simulink model "rectifiers01"  (R2020b)
settings: Solver=VariableStepAuto  StartTime=0.0  StopTime=2/60  RelTol=1e-3
InitFcn:
  | R = 1;
libraries: fl_lib x61, ee_lib x29, nesl_utility x28, powerlib x1
settings Model: Creator=gdudgeon  LastModifiedBy=gdudgeon
settings DataIOCC: SaveOutput=off  DSMLogging=off  InspectSignalLogs=on  SaveTime=off  ReturnWorkspaceOutputs=off

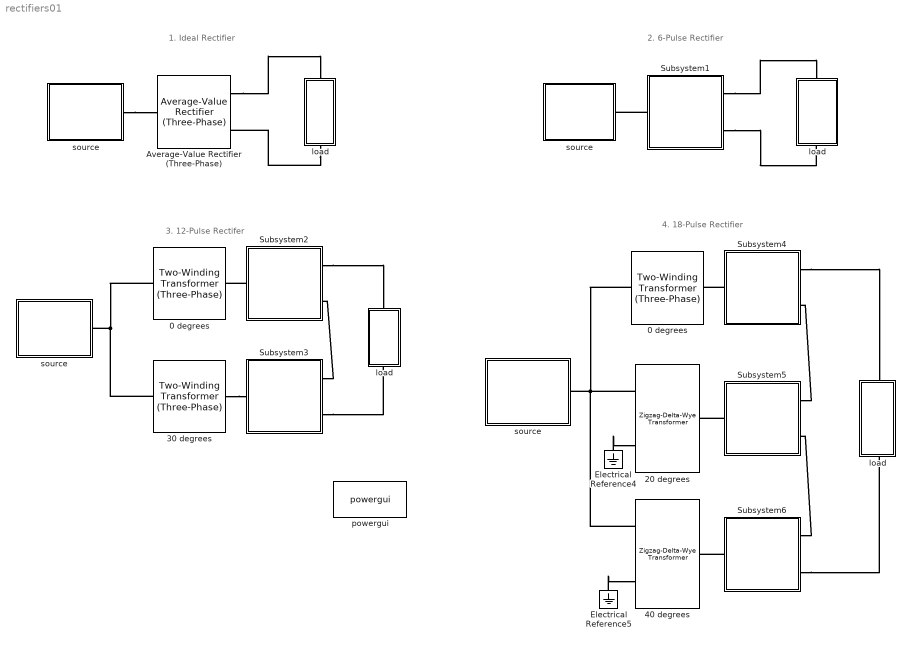
== system rectifiers01 ==
  note: 4. 18-Pulse Rectifier
  note: 3. 12-Pulse Rectifer
  note: 2. 6-Pulse Rectifier
  note: 1. Ideal Rectifier
  " load" : Subsystem
      settings: PortSchema="{\"entries\":[{\"content\":{\"sides\":[{\"content\":{\"connectorIds\":[]},\"type\":\"ConnectorPlacement.EquallySpacedRectSide\",\"uuid\":\"d22d21fe-0203-4dc0-90b3-23bdd03d5351\"},{\"content\":{\"connectorIds\":[],\"side\":\"RIGHT\"},\"type\":\"ConnectorPlacement.EquallySpacedRectSide\",\"uuid\":\"b0134291-2b85-4d9d-ab7a-f2a22f0cc825\"},{\"content\":{\"connectorIds\":[\"LConn1\"],\"side\":\"TOP\"},\"type\":\"ConnectorPlacement.EquallySpacedRectSide\",\"uuid\":\"0f25709f-cbaa-4d6a-91aa-03a240b6065b\"},{\"content\":{\"connectorIds\":[\"RConn1\"],\"side\":\"BOTTOM\"},\"type\":\"ConnectorPlacement.EquallySpacedRectSide\",\"uuid\":\"1cb50f91-b6f6-42a0-b153-9b586f859798\"},{\"content\":{\"connectorIds\":[],\"side\":\"HIDDEN\"},\"type\":\"ConnectorPlacement.EquallySpacedRectSide\",\"uuid\":\"613bd7c7-2abb-4a7f-9569-314c864fd2f9\"}]},\"type\":\"ConnectorPlacement.EquallySpacedConnector\",\"uuid\":\"0347b9d2-0f82-406a-989b-2d0201140953\"}],\"packageUris\":[\"http://schema.mathworks.com/mf0/Connector/R2020b\"],\"version\":\"1.0\"}"
  " source" : Subsystem
  0 degrees : ee_lib/Passive/Transformers/Two-Winding Transformer (Three-Phase)  SRated=100e3 V*A  FRated=60 Hz  Winding1Connection=ee.enum.windingconnection.Y  VRated1=sqrt(3) * 100 / sqrt(2) V  Winding2Connection=ee.enum.windingconnection.Y  VRated2=sqrt(3) * 50 / sqrt(2) V  CoreType=ee.enum.coretype.threelimb  pu_Rw1=0.01e-3  pu_Xl1=0.001e-3  pu_Rw2=0.01e-3  pu_Xl2=0.001e-3  pu_Rm=50000  saturation_option=ee.enum.transformer_saturation.exclude  pu_Xm=50000  current_data=[0, .002, 1, 2]  magnetic_flux_data=[0, 1.2, 1.5, 1.51]  pu_X0=0.5  i1_specify=off  i1_priority=None  i1=[ 0 0 0 ] A  i1_nominal_specify=off  i1_nominal_unit=A  i1_nominal_value=1  i2_specify=off  i2_priority=None  i2=[ 0 0 0 ] A  i2_nominal_specify=off  i2_nominal_unit=A  i2_nominal_value=1  phi_specify=off  phi_priority=None  phi=[ 0 0 0 ]  phi_nominal_specify=off  phi_nominal_unit=1  phi_nominal_value=1  power_dissipated_specify=off  power_dissipated_priority=None  power_dissipated=0 W  power_dissipated_nominal_specify=off  power_dissipated_nominal_unit=W  power_dissipated_nominal_value=1
      settings: SourceProductBaseCode=PS  InternalSimscapePortConfiguration="{\"Bottom\":[],\"Left\":[{\"id\":\"N1\",\"label\":\"~1\",\"type\":\"foundation.electrical.three_phase\"}],\"Right\":[{\"id\":\"N2\",\"label\":\"~2\",\"type\":\"foundation.electrical.three_phase\"}],\"Top\":[]}"
  "0 degrees " : ee_lib/Passive/Transformers/Two-Winding Transformer (Three-Phase)  SRated=100e3 V*A  FRated=60 Hz  Winding1Connection=ee.enum.windingconnection.Y  VRated1=sqrt(3) * 100 / sqrt(2) V  Winding2Connection=ee.enum.windingconnection.Y  VRated2=sqrt(3) * 33.3 / sqrt(2) V  CoreType=ee.enum.coretype.threelimb  pu_Rw1=0.01e-3  pu_Xl1=0.001e-3  pu_Rw2=0.01e-3  pu_Xl2=0.001e-3  pu_Rm=50000  saturation_option=ee.enum.transformer_saturation.exclude  pu_Xm=50000  current_data=[0, .002, 1, 2]  magnetic_flux_data=[0, 1.2, 1.5, 1.51]  pu_X0=0.5  i1_specify=off  i1_priority=None  i1=[ 0 0 0 ] A  i1_nominal_specify=off  i1_nominal_unit=A  i1_nominal_value=1  i2_specify=off  i2_priority=None  i2=[ 0 0 0 ] A  i2_nominal_specify=off  i2_nominal_unit=A  i2_nominal_value=1  phi_specify=off  phi_priority=None  phi=[ 0 0 0 ]  phi_nominal_specify=off  phi_nominal_unit=1  phi_nominal_value=1  power_dissipated_specify=off  power_dissipated_priority=None  power_dissipated=0 W  power_dissipated_nominal_specify=off  power_dissipated_nominal_unit=W  power_dissipated_nominal_value=1
      settings: SourceProductBaseCode=PS  InternalSimscapePortConfiguration="{\"Bottom\":[],\"Left\":[{\"id\":\"N1\",\"label\":\"~1\",\"type\":\"foundation.electrical.three_phase\"}],\"Right\":[{\"id\":\"N2\",\"label\":\"~2\",\"type\":\"foundation.electrical.three_phase\"}],\"Top\":[]}"
  20 degrees : ee_lib/Passive/Transformers/Zigzag-Delta-Wye Transformer  SRated=100e3 V*A  FRated=60 Hz  VRated1=sqrt(3) * 33.3 / sqrt(2) V  interconnection_option=ee.enum.zigzaginterconnection.floatingNeutral  configuration_option=ee.enum.zigzagconfiguration.Wye  pu_Rw1=0.01e-3  pu_Xl1=0.001e-3  pu_Rm=50000  saturation_option=ee.enum.transformer_saturation.exclude  deltaconnection_option=ee.enum.deltaconnection.delta1  VRated2=sqrt(3) * 50 / sqrt(2) V  magnetic_flux_data=[0, 1.2, 1.5, 1.51]  pu_Rw2=0.01  pu_Xl2=0.001  VRated3=sqrt(3) * 100 / sqrt(2) V  pu_Rw3=0.01e-3  pu_Xl3=0.001e-3  pu_Xm=50000  current_data=[0, .002, 1, 2]  phaseShift=20 deg  i1_specify=off  i1_priority=None  i1=[ 0 0 0 ] A  i1_nominal_specify=off  i1_nominal_unit=A  i1_nominal_value=1  i2_specify=off  i2_priority=None  i2=[ 0 0 0 ] A  i2_nominal_specify=off  i2_nominal_unit=A  i2_nominal_value=1  i3_specify=off  i3_priority=None  i3=[ 0 0 0 ] A  i3_nominal_specify=off  i3_nominal_unit=A  i3_nominal_value=1  phi_specify=off  phi_priority=None  phi=[ 0 0 0 ]  phi_nominal_specify=off  phi_nominal_unit=1  phi_nominal_value=1  phaseShift_increment=0.1 deg
      settings: SourceProductBaseCode=PS  InternalSimscapePortConfiguration="{\"Bottom\":[],\"Left\":[{\"id\":\"N1\",\"label\":\"~1\",\"type\":\"foundation.electrical.three_phase\"}],\"Right\":[{\"id\":\"N3\",\"label\":\"~3\",\"type\":\"foundation.electrical.three_phase\"},{\"id\":\"n3\",\"label\":\"n3\",\"type\":\"foundation.electrical.electrical\"}],\"Top\":[]}"
  30 degrees : ee_lib/Passive/Transformers/Two-Winding Transformer (Three-Phase)  SRated=100e3 V*A  FRated=60 Hz  Winding1Connection=ee.enum.windingconnection.delta1  VRated1=sqrt(3) * 100 / sqrt(2) V  Winding2Connection=ee.enum.windingconnection.Y  VRated2=sqrt(3) * 50 / sqrt(2) V  CoreType=ee.enum.coretype.threelimb  pu_Rw1=0.01e-3  pu_Xl1=0.001e-3  pu_Rw2=0.01e-3  pu_Xl2=0.001e-3  pu_Rm=50000  saturation_option=ee.enum.transformer_saturation.exclude  pu_Xm=50000  current_data=[0, .002, 1, 2]  magnetic_flux_data=[0, 1.2, 1.5, 1.51]  pu_X0=0.5  i1_specify=off  i1_priority=None  i1=[ 0 0 0 ] A  i1_nominal_specify=off  i1_nominal_unit=A  i1_nominal_value=1  i2_specify=off  i2_priority=None  i2=[ 0 0 0 ] A  i2_nominal_specify=off  i2_nominal_unit=A  i2_nominal_value=1  phi_specify=off  phi_priority=None  phi=[ 0 0 0 ]  phi_nominal_specify=off  phi_nominal_unit=1  phi_nominal_value=1  power_dissipated_specify=off  power_dissipated_priority=None  power_dissipated=0 W  power_dissipated_nominal_specify=off  power_dissipated_nominal_unit=W  power_dissipated_nominal_value=1
      settings: SourceProductBaseCode=PS  InternalSimscapePortConfiguration="{\"Bottom\":[],\"Left\":[{\"id\":\"N1\",\"label\":\"~1\",\"type\":\"foundation.electrical.three_phase\"}],\"Right\":[{\"id\":\"N2\",\"label\":\"~2\",\"type\":\"foundation.electrical.three_phase\"}],\"Top\":[]}"
  40 degrees : ee_lib/Passive/Transformers/Zigzag-Delta-Wye Transformer  SRated=100e3 V*A  FRated=60 Hz  VRated1=sqrt(3) * 33.3 / sqrt(2) V  interconnection_option=ee.enum.zigzaginterconnection.floatingNeutral  configuration_option=ee.enum.zigzagconfiguration.Wye  pu_Rw1=0.01e-3  pu_Xl1=0.001e-3  pu_Rm=50000  saturation_option=ee.enum.transformer_saturation.exclude  deltaconnection_option=ee.enum.deltaconnection.delta1  VRated2=sqrt(3) * 50 / sqrt(2) V  magnetic_flux_data=[0, 1.2, 1.5, 1.51]  pu_Rw2=0.01  pu_Xl2=0.001  VRated3=sqrt(3) * 100 / sqrt(2) V  pu_Rw3=0.01e-3  pu_Xl3=0.001e-3  pu_Xm=50000  current_data=[0, .002, 1, 2]  phaseShift=40 deg  i1_specify=off  i1_priority=None  i1=[ 0 0 0 ] A  i1_nominal_specify=off  i1_nominal_unit=A  i1_nominal_value=1  i2_specify=off  i2_priority=None  i2=[ 0 0 0 ] A  i2_nominal_specify=off  i2_nominal_unit=A  i2_nominal_value=1  i3_specify=off  i3_priority=None  i3=[ 0 0 0 ] A  i3_nominal_specify=off  i3_nominal_unit=A  i3_nominal_value=1  phi_specify=off  phi_priority=None  phi=[ 0 0 0 ]  phi_nominal_specify=off  phi_nominal_unit=1  phi_nominal_value=1  phaseShift_increment=0.1 deg
      settings: SourceProductBaseCode=PS  InternalSimscapePortConfiguration="{\"Bottom\":[],\"Left\":[{\"id\":\"N1\",\"label\":\"~1\",\"type\":\"foundation.electrical.three_phase\"}],\"Right\":[{\"id\":\"N3\",\"label\":\"~3\",\"type\":\"foundation.electrical.three_phase\"},{\"id\":\"n3\",\"label\":\"n3\",\"type\":\"foundation.electrical.electrical\"}],\"Top\":[]}"
  Average-Value Rectifier (Three-Phase) : ee_lib/Semiconductors & Converters/Converters/Average-Value Rectifier (Three-Phase)  VRated=4160 V  Pfixed=1e3 W
      settings: SourceProductBaseCode=PS  InternalSimscapePortConfiguration="{\"Bottom\":[],\"Left\":[{\"id\":\"N\",\"label\":\"~\",\"type\":\"foundation.electrical.three_phase\"}],\"Right\":[{\"id\":\"p\",\"label\":\"+\",\"type\":\"foundation.electrical.electrical\"},{\"id\":\"n\",\"label\":\"-\",\"type\":\"foundation.electrical.electrical\"}],\"Top\":[]}"
  Electrical Reference4 : fl_lib/Electrical/Electrical Elements/Electrical Reference
  Electrical Reference5 : fl_lib/Electrical/Electrical Elements/Electrical Reference
  Subsystem1 : Subsystem
      mask Display: image('diode.jpg')
  Subsystem2 : Subsystem
      mask Display: image('diode.jpg')
  Subsystem3 : Subsystem
      mask Display: image('diode.jpg')
  Subsystem4 : Subsystem
      mask Display: image('diode.jpg')
  Subsystem5 : Subsystem
      mask Display: image('diode.jpg')
  Subsystem6 : Subsystem
      mask Display: image('diode.jpg')
  load : Subsystem
      settings: PortSchema="{\"entries\":[{\"content\":{\"sides\":[{\"content\":{\"connectorIds\":[]},\"type\":\"ConnectorPlacement.EquallySpacedRectSide\",\"uuid\":\"d22d21fe-0203-4dc0-90b3-23bdd03d5351\"},{\"content\":{\"connectorIds\":[],\"side\":\"RIGHT\"},\"type\":\"ConnectorPlacement.EquallySpacedRectSide\",\"uuid\":\"b0134291-2b85-4d9d-ab7a-f2a22f0cc825\"},{\"content\":{\"connectorIds\":[\"LConn1\"],\"side\":\"TOP\"},\"type\":\"ConnectorPlacement.EquallySpacedRectSide\",\"uuid\":\"0f25709f-cbaa-4d6a-91aa-03a240b6065b\"},{\"content\":{\"connectorIds\":[\"RConn1\"],\"side\":\"BOTTOM\"},\"type\":\"ConnectorPlacement.EquallySpacedRectSide\",\"uuid\":\"adaf0646-c50e-4c15-9e13-216df2ff67a6\"},{\"content\":{\"connectorIds\":[],\"side\":\"HIDDEN\"},\"type\":\"ConnectorPlacement.EquallySpacedRectSide\",\"uuid\":\"613bd7c7-2abb-4a7f-9569-314c864fd2f9\"}]},\"type\":\"ConnectorPlacement.EquallySpacedConnector\",\"uuid\":\"0347b9d2-0f82-406a-989b-2d0201140953\"}],\"packageUris\":[\"http://schema.mathworks.com/mf0/Connector/R2020b\"],\"version\":\"1.0\"}"
  "load " : Subsystem
      settings: PortSchema="{\"entries\":[{\"content\":{\"sides\":[{\"content\":{\"connectorIds\":[]},\"type\":\"ConnectorPlacement.EquallySpacedRectSide\",\"uuid\":\"d22d21fe-0203-4dc0-90b3-23bdd03d5351\"},{\"content\":{\"connectorIds\":[],\"side\":\"RIGHT\"},\"type\":\"ConnectorPlacement.EquallySpacedRectSide\",\"uuid\":\"b0134291-2b85-4d9d-ab7a-f2a22f0cc825\"},{\"content\":{\"connectorIds\":[\"LConn1\"],\"side\":\"TOP\"},\"type\":\"ConnectorPlacement.EquallySpacedRectSide\",\"uuid\":\"0f25709f-cbaa-4d6a-91aa-03a240b6065b\"},{\"content\":{\"connectorIds\":[\"RConn1\"],\"side\":\"BOTTOM\"},\"type\":\"ConnectorPlacement.EquallySpacedRectSide\",\"uuid\":\"28ce9175-6449-4b65-9253-b55dcacbce87\"},{\"content\":{\"connectorIds\":[],\"side\":\"HIDDEN\"},\"type\":\"ConnectorPlacement.EquallySpacedRectSide\",\"uuid\":\"613bd7c7-2abb-4a7f-9569-314c864fd2f9\"}]},\"type\":\"ConnectorPlacement.EquallySpacedConnector\",\"uuid\":\"0347b9d2-0f82-406a-989b-2d0201140953\"}],\"packageUris\":[\"http://schema.mathworks.com/mf0/Connector/R2020b\"],\"version\":\"1.0\"}"
  "load  " : Subsystem
      settings: PortSchema="{\"entries\":[{\"content\":{\"sides\":[{\"content\":{\"connectorIds\":[]},\"type\":\"ConnectorPlacement.EquallySpacedRectSide\",\"uuid\":\"d22d21fe-0203-4dc0-90b3-23bdd03d5351\"},{\"content\":{\"connectorIds\":[],\"side\":\"RIGHT\"},\"type\":\"ConnectorPlacement.EquallySpacedRectSide\",\"uuid\":\"b0134291-2b85-4d9d-ab7a-f2a22f0cc825\"},{\"content\":{\"connectorIds\":[\"LConn1\"],\"side\":\"TOP\"},\"type\":\"ConnectorPlacement.EquallySpacedRectSide\",\"uuid\":\"0f25709f-cbaa-4d6a-91aa-03a240b6065b\"},{\"content\":{\"connectorIds\":[\"RConn1\"],\"side\":\"BOTTOM\"},\"type\":\"ConnectorPlacement.EquallySpacedRectSide\",\"uuid\":\"e9fa62c1-7df6-4db7-8279-90334c7dd692\"},{\"content\":{\"connectorIds\":[],\"side\":\"HIDDEN\"},\"type\":\"ConnectorPlacement.EquallySpacedRectSide\",\"uuid\":\"613bd7c7-2abb-4a7f-9569-314c864fd2f9\"}]},\"type\":\"ConnectorPlacement.EquallySpacedConnector\",\"uuid\":\"0347b9d2-0f82-406a-989b-2d0201140953\"}],\"packageUris\":[\"http://schema.mathworks.com/mf0/Connector/R2020b\"],\"version\":\"1.0\"}"
  powergui : powerlib/powergui  Priority=1  SimulationMode=Continuous  SampleTime=50e-6  frequency=60  Iterations=50  frequencyindice=60  Pbase=100e6  ErrMax=1e-4  UnitsV=kV  UnitsW=MW  buscounter=0  FunctionMessages=off  echomessages=off  EnableUseOfTLC=off  CurrentSourceSwitches=off  DisableSnubberDevices=off  DisableRonSwitches=off  DisableVfSwitches=off  DisplayEquations=off  AutomaticDiscreteSolvers=off  SolverType=Tustin/Backward Euler (TBE)  Interpol=off  ExternalGateDelay=off  methode=off  Ts=100  x0status=blocks  SPID=on  SwTol=0  HookPort=off  NonlinearTolerance=1e-4  nMaxIteration=100  ContinueOnMaxIteration=off  RestoreLinks=warning  ResistiveCurrentMeasurement=off  Frange=[0:2:500]  Ylog=off  Xlog=on  ShowGrid=off  save=off  variable=ZData  structure=logsout  ZoomFFT=off  StartTime=0.01  cycles=1  DisplayStyle=1  fundamental=60  FreqAxis=on  MaxFrequency=2000  frequencyindicesteady=1  RmsSteady=1  display=off
  source : Subsystem
  "source " : Subsystem
  "source  " : Subsystem
  connections:
  Subsystem3/LConn1 -- Subsystem2/LConn2
  30 degrees/RConn1 -- Subsystem3/RConn1
  Subsystem2/RConn1 -- 0 degrees/RConn1
  Subsystem4/RConn1 -- "0 degrees "/RConn1
  Subsystem5/LConn1 -- Subsystem4/LConn2
  Subsystem5/RConn1 -- 20 degrees/LConn1
  Electrical Reference4/LConn1 -- 20 degrees/RConn2
  Subsystem6/RConn1 -- 40 degrees/LConn1
  Electrical Reference5/LConn1 -- 40 degrees/RConn2
  Subsystem6/LConn1 -- Subsystem5/LConn2
  source/RConn1 -- Average-Value Rectifier (Three-Phase)/LConn1
  Average-Value Rectifier (Three-Phase)/RConn1 -- load/LConn1
  load/RConn1 -- Average-Value Rectifier (Three-Phase)/RConn2
  Subsystem2/LConn1 -- "load "/LConn1
  Subsystem3/LConn2 -- "load "/RConn1
  0 degrees/LConn1 -- 30 degrees/LConn1 -- "source "/RConn1
  Subsystem1/RConn1 -- "source  "/RConn1
  Subsystem1/LConn1 -- "load  "/LConn1
  Subsystem1/LConn2 -- "load  "/RConn1
  20 degrees/RConn1 -- "0 degrees "/LConn1 -- 40 degrees/RConn1 -- " source"/RConn1
  Subsystem4/LConn1 -- " load"/LConn1
  Subsystem6/LConn2 -- " load"/RConn1

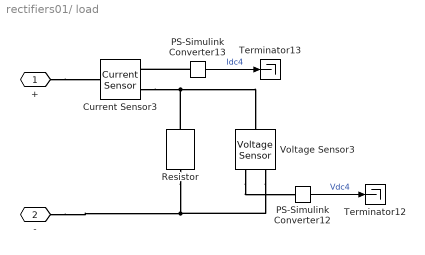
== system rectifiers01/ load ==
  Current Sensor3 : fl_lib/Electrical/Electrical Sensors/Current Sensor
  PS-Simulink Converter12 : nesl_utility/PS-Simulink Converter  PhysicalDomain=network_engine_domain  SubClassName=ps_output  LeftPortType=input  RightPortType=output  PseudoPeriodic=off  Frequencies=[]  Unit=inherit  AffineConversion=off
  PS-Simulink Converter13 : nesl_utility/PS-Simulink Converter  PhysicalDomain=network_engine_domain  SubClassName=ps_output  LeftPortType=input  RightPortType=output  PseudoPeriodic=off  Frequencies=[]  Unit=inherit  AffineConversion=off
  Resistor : fl_lib/Electrical/Electrical Elements/Resistor  R=R Ohm  i_specify=off  i_priority=None  i=0 A  i_nominal_specify=off  i_nominal_unit=A  i_nominal_value=1  v_specify=off  v_priority=None  v=0 V  v_nominal_specify=off  v_nominal_unit=V  v_nominal_value=1
  Terminator12 : Terminator
  Terminator13 : Terminator
  Voltage Sensor3 : fl_lib/Electrical/Electrical Sensors/Voltage Sensor
  + : PMIOPort  Side=Left
  - : PMIOPort  Port=2  Side=Right
  wires:
  PS-Simulink Converter13/1 -> Terminator13/1  "Idc4"
  PS-Simulink Converter12/1 -> Terminator12/1  "Vdc4"
  connections:
  +/RConn1 -- Current Sensor3/LConn1
  Voltage Sensor3/RConn1 -- PS-Simulink Converter12/LConn1
  Current Sensor3/RConn2 -- Resistor/LConn1 -- Voltage Sensor3/LConn1
  PS-Simulink Converter13/LConn1 -- Current Sensor3/RConn1
  Voltage Sensor3/RConn2 -- Resistor/RConn1 -- -/RConn1

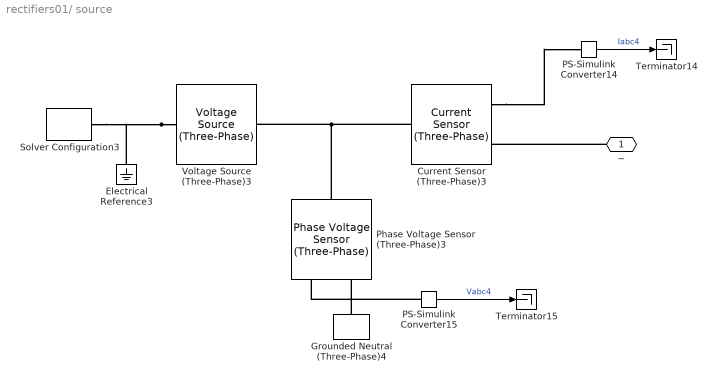
== system rectifiers01/ source ==
  Current Sensor (Three-Phase)3 : ee_lib/Sensors & Transducers/Current Sensor (Three-Phase)
  Electrical Reference3 : fl_lib/Electrical/Electrical Elements/Electrical Reference
  Grounded Neutral (Three-Phase)4 : ee_lib/Connectors & References/Grounded Neutral (Three-Phase)
      settings: SourceProductBaseCode=PS
  PS-Simulink Converter14 : nesl_utility/PS-Simulink Converter  PhysicalDomain=network_engine_domain  SubClassName=ps_output  LeftPortType=input  RightPortType=output  PseudoPeriodic=off  Frequencies=[]  Unit=inherit  AffineConversion=off
  PS-Simulink Converter15 : nesl_utility/PS-Simulink Converter  PhysicalDomain=network_engine_domain  SubClassName=ps_output  LeftPortType=input  RightPortType=output  PseudoPeriodic=off  Frequencies=[]  Unit=inherit  AffineConversion=off
  Phase Voltage Sensor (Three-Phase)3 : ee_lib/Sensors & Transducers/Phase Voltage Sensor (Three-Phase)
      settings: SourceProductBaseCode=PS
  Solver Configuration3 : nesl_utility/Solver Configuration  PhysicalDomain=network_engine_domain  SubClassName=solver  LeftPortType=input  RightPortType=generic  Tones=[]  Harmonics=[]  SimulateNoise=off  Profile=off  UseLocalSampling=off  EnableSwitchedLinearOptims=on  FrequencyDomain=off  UseCCode=off  RelTol=0.001  AbsTol=1e-06  MinStep=1e-09  ToWorkspace=off  RevertToSquareIcSolve=off  NumHomotopyIterations=100  PhasorMode=off  PhasorModeNumHarmonics=1  DoDC=off  ResidualTolerance=1e-09  UseLocalSolver=on  LocalSolverChoice=NE_BACKWARD_EULER_ADVANCER  LocalSolverSampleTime=50e-6  DoFixedCost=on  MaxNonlinIter=3  MaxModeIter=2  ComputeImpulses=off  ImpulseIterations=2  LinearAlgebra=auto  EquationFormulation=NE_TIME_EF  DelaysMemoryBudget=1024  AutomaticFiltering=on  FilteringTimeConstant=0.001  PartitionStorageMethod=AS_NEEDED  PartitionMemoryBudget=1024  PartitionMethod=ROBUST
  Terminator14 : Terminator
  Terminator15 : Terminator
  Voltage Source (Three-Phase)3 : ee_lib/Sources/Voltage Source (Three-Phase)  vline_rms=sqrt(3) * 100 / sqrt(2) V  shift=0 deg  freq=60 Hz  impedance_option=0  SShortCircuit=1e6 V*A  XR=15  R=0.01 Ohm  L=3.97e-4 H  G_parasitic=0 1/Ohm  harmonic_option=0  harmonic_orders=[5, 7, 11, 13]  harmonic_ratios=[.1, .1, .1, .1]  I_specify=off  I_priority=None  I=[ 0 0 0 ] A  I_nominal_specify=off  I_nominal_unit=A  I_nominal_value=1
      settings: SourceProductBaseCode=PS
  ~ : PMIOPort  Side=Right
  wires:
  PS-Simulink Converter15/1 -> Terminator15/1  "Vabc4"
  PS-Simulink Converter14/1 -> Terminator14/1  "Iabc4"
  connections:
  Grounded Neutral (Three-Phase)4/LConn1 -- Phase Voltage Sensor (Three-Phase)3/RConn2
  Current Sensor (Three-Phase)3/RConn1 -- PS-Simulink Converter14/LConn1
  Phase Voltage Sensor (Three-Phase)3/LConn1 -- Current Sensor (Three-Phase)3/LConn1 -- Voltage Source (Three-Phase)3/RConn1
  PS-Simulink Converter15/LConn1 -- Phase Voltage Sensor (Three-Phase)3/RConn1
  Voltage Source (Three-Phase)3/LConn1 -- Electrical Reference3/LConn1 -- Solver Configuration3/RConn1
  ~/RConn1 -- Current Sensor (Three-Phase)3/RConn2

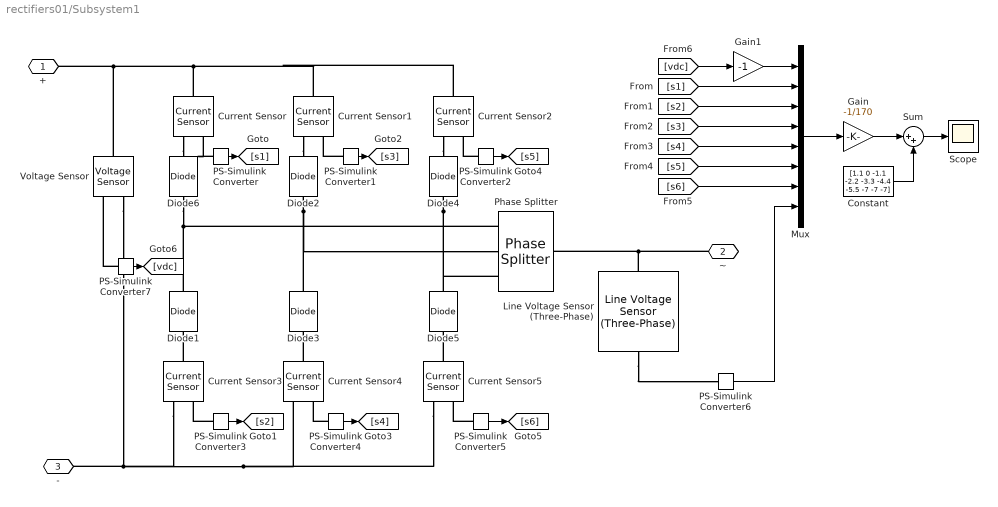
== system rectifiers01/Subsystem1 ==
  Constant : Constant  Value=[1.1 0 -1.1 -2.2 -3.3 -4.4 -5.5 -7 -7 -7]
  Current Sensor{,1..5} (6 alike) : fl_lib/Electrical/Electrical Sensors/Current Sensor
  Diode{1..6} (6 alike) : fl_lib/Electrical/Electrical Elements/Diode  Vf=0.6 V  Ron=1e-5 Ohm  Goff=1e-8 1/Ohm  i_specify=off  i_priority=None  i=0 A  i_nominal_specify=off  i_nominal_unit=A  i_nominal_value=1  v_specify=off  v_priority=None  v=0 V  v_nominal_specify=off  v_nominal_unit=V  v_nominal_value=1
  Gain : Gain  Gain=-1/170
  Gain1 : Gain  Gain=-1
  Line Voltage Sensor (Three-Phase) : ee_lib/Sensors & Transducers/Line Voltage Sensor (Three-Phase)
      settings: SourceProductBaseCode=PS
  Mux : Mux  Inputs=8
  PS-Simulink Converter{,1..7} (8 alike) : nesl_utility/PS-Simulink Converter  PhysicalDomain=network_engine_domain  SubClassName=ps_output  LeftPortType=input  RightPortType=output  PseudoPeriodic=off  Frequencies=[]  Unit=inherit  AffineConversion=off
  Phase Splitter : ee_lib/Connectors & References/Phase Splitter
      settings: SourceProductBaseCode=PS
  Scope : Scope
  Sum : Sum  Inputs=|++
  Voltage Sensor : fl_lib/Electrical/Electrical Sensors/Voltage Sensor
  + : PMIOPort  Side=Left
  ~ : PMIOPort  Port=2  Side=Right
  - : PMIOPort  Port=3  Side=Left
  wires:
  PS-Simulink Converter/1 -> [s1]
  PS-Simulink Converter3/1 -> [s2]
  PS-Simulink Converter1/1 -> [s3]
  PS-Simulink Converter4/1 -> [s4]
  PS-Simulink Converter2/1 -> [s5]
  PS-Simulink Converter5/1 -> [s6]
  Mux/1 -> Gain/1
  Gain/1 -> Sum/1
  Sum/1 -> Scope/1
  Constant/1 -> Sum/2
  PS-Simulink Converter6/1 -> Mux/8
  PS-Simulink Converter7/1 -> [vdc]
  [vdc] -> Gain1/1
  [s1] -> Mux/2
  [s2] -> Mux/3
  [s3] -> Mux/4
  [s4] -> Mux/5
  [s5] -> Mux/6
  [s6] -> Mux/7
  Gain1/1 -> Mux/1
  connections:
  Diode4/LConn1 -- Phase Splitter/RConn3 -- Diode5/RConn1
  Current Sensor5/RConn2 -- Current Sensor4/RConn2 -- Current Sensor3/RConn2 -- Voltage Sensor/RConn2 -- -/RConn1
  Diode6/LConn1 -- Diode1/RConn1 -- Phase Splitter/RConn1
  Diode2/LConn1 -- Diode3/RConn1 -- Phase Splitter/RConn2
  ~/RConn1 -- Line Voltage Sensor (Three-Phase)/LConn1 -- Phase Splitter/LConn1
  Current Sensor2/LConn1 -- Current Sensor1/LConn1 -- Current Sensor/LConn1 -- Voltage Sensor/LConn1 -- +/RConn1
  Current Sensor/RConn2 -- Diode6/RConn1
  Current Sensor1/RConn2 -- Diode2/RConn1
  Current Sensor2/RConn2 -- Diode4/RConn1
  Current Sensor3/LConn1 -- Diode1/LConn1
  Current Sensor4/LConn1 -- Diode3/LConn1
  Current Sensor5/LConn1 -- Diode5/LConn1
  PS-Simulink Converter/LConn1 -- Current Sensor/RConn1
  PS-Simulink Converter1/LConn1 -- Current Sensor1/RConn1
  PS-Simulink Converter2/LConn1 -- Current Sensor2/RConn1
  PS-Simulink Converter3/LConn1 -- Current Sensor3/RConn1
  PS-Simulink Converter4/LConn1 -- Current Sensor4/RConn1
  PS-Simulink Converter5/LConn1 -- Current Sensor5/RConn1
  Line Voltage Sensor (Three-Phase)/RConn1 -- PS-Simulink Converter6/LConn1
  PS-Simulink Converter7/LConn1 -- Voltage Sensor/RConn1

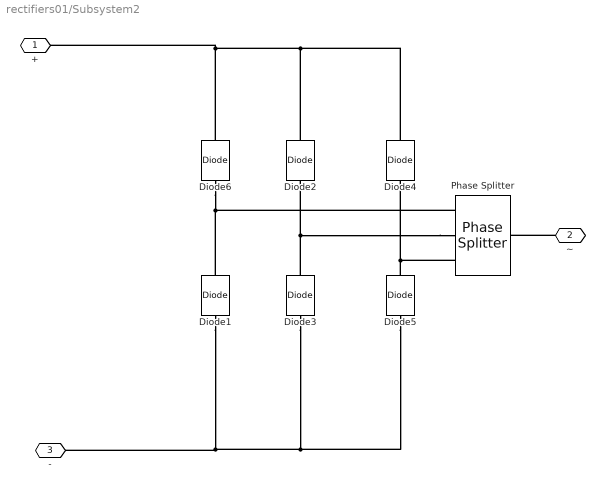
== system rectifiers01/Subsystem2 ==
  Diode{1..6} (6 alike) : fl_lib/Electrical/Electrical Elements/Diode  Vf=0.6 V  Ron=1e-5 Ohm  Goff=1e-8 1/Ohm  i_specify=off  i_priority=None  i=0 A  i_nominal_specify=off  i_nominal_unit=A  i_nominal_value=1  v_specify=off  v_priority=None  v=0 V  v_nominal_specify=off  v_nominal_unit=V  v_nominal_value=1
  Phase Splitter : ee_lib/Connectors & References/Phase Splitter
      settings: SourceProductBaseCode=PS
  + : PMIOPort  Side=Left
  ~ : PMIOPort  Port=2  Side=Right
  - : PMIOPort  Port=3  Side=Left
  connections:
  Diode6/RConn1 -- +/RConn1 -- Diode4/RConn1 -- Diode2/RConn1
  ~/RConn1 -- Phase Splitter/LConn1
  Phase Splitter/RConn2 -- Diode3/RConn1 -- Diode2/LConn1
  Diode1/RConn1 -- Phase Splitter/RConn1 -- Diode6/LConn1
  Diode1/LConn1 -- Diode5/LConn1 -- Diode3/LConn1 -- -/RConn1
  Phase Splitter/RConn3 -- Diode5/RConn1 -- Diode4/LConn1

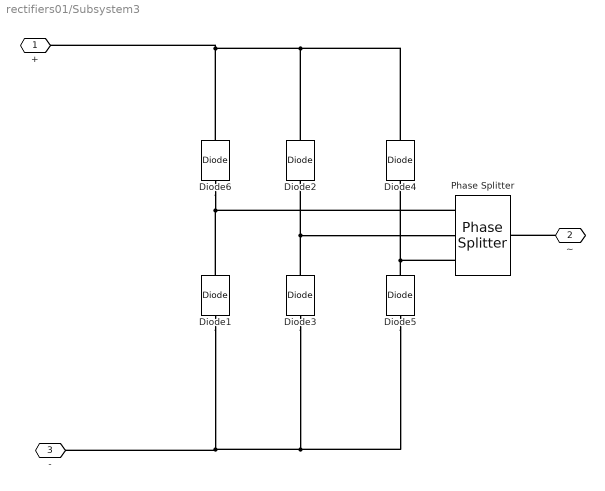
== system rectifiers01/Subsystem3 ==
  Diode{1..6} (6 alike) : fl_lib/Electrical/Electrical Elements/Diode  Vf=0.6 V  Ron=1e-5 Ohm  Goff=1e-8 1/Ohm  i_specify=off  i_priority=None  i=0 A  i_nominal_specify=off  i_nominal_unit=A  i_nominal_value=1  v_specify=off  v_priority=None  v=0 V  v_nominal_specify=off  v_nominal_unit=V  v_nominal_value=1
  Phase Splitter : ee_lib/Connectors & References/Phase Splitter
      settings: SourceProductBaseCode=PS
  + : PMIOPort  Side=Left
  ~ : PMIOPort  Port=2  Side=Right
  - : PMIOPort  Port=3  Side=Left
  connections:
  Diode4/LConn1 -- Diode5/RConn1 -- Phase Splitter/RConn3
  -/RConn1 -- Diode3/LConn1 -- Diode5/LConn1 -- Diode1/LConn1
  Diode6/LConn1 -- Phase Splitter/RConn1 -- Diode1/RConn1
  Diode2/LConn1 -- Diode3/RConn1 -- Phase Splitter/RConn2
  ~/RConn1 -- Phase Splitter/LConn1
  Diode2/RConn1 -- Diode4/RConn1 -- +/RConn1 -- Diode6/RConn1

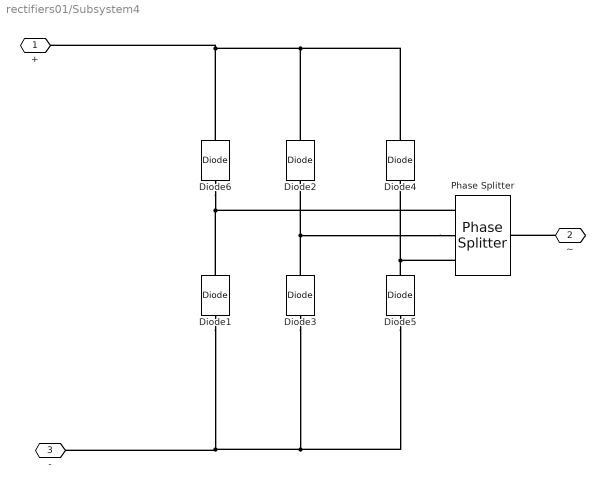
== system rectifiers01/Subsystem4 ==
  Diode{1..6} (6 alike) : fl_lib/Electrical/Electrical Elements/Diode  Vf=0.6 V  Ron=1e-5 Ohm  Goff=1e-8 1/Ohm  i_specify=off  i_priority=None  i=0 A  i_nominal_specify=off  i_nominal_unit=A  i_nominal_value=1  v_specify=off  v_priority=None  v=0 V  v_nominal_specify=off  v_nominal_unit=V  v_nominal_value=1
  Phase Splitter : ee_lib/Connectors & References/Phase Splitter
      settings: SourceProductBaseCode=PS
  + : PMIOPort  Side=Left
  ~ : PMIOPort  Port=2  Side=Right
  - : PMIOPort  Port=3  Side=Left
  connections:
  Diode6/RConn1 -- +/RConn1 -- Diode4/RConn1 -- Diode2/RConn1
  ~/RConn1 -- Phase Splitter/LConn1
  Phase Splitter/RConn2 -- Diode3/RConn1 -- Diode2/LConn1
  Diode1/RConn1 -- Phase Splitter/RConn1 -- Diode6/LConn1
  Diode1/LConn1 -- Diode5/LConn1 -- Diode3/LConn1 -- -/RConn1
  Phase Splitter/RConn3 -- Diode5/RConn1 -- Diode4/LConn1

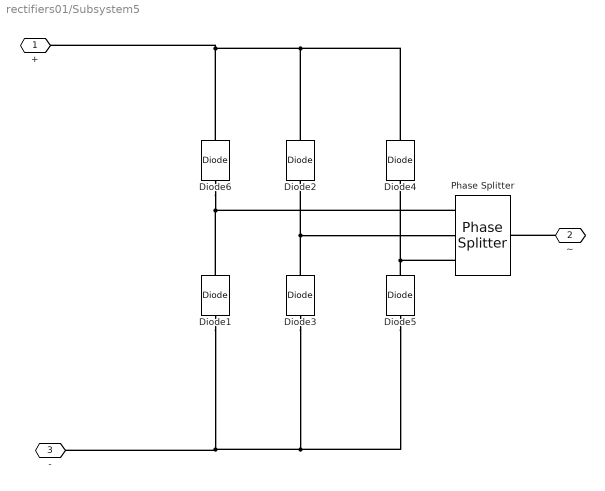
== system rectifiers01/Subsystem5 ==
  Diode{1..6} (6 alike) : fl_lib/Electrical/Electrical Elements/Diode  Vf=0.6 V  Ron=1e-5 Ohm  Goff=1e-8 1/Ohm  i_specify=off  i_priority=None  i=0 A  i_nominal_specify=off  i_nominal_unit=A  i_nominal_value=1  v_specify=off  v_priority=None  v=0 V  v_nominal_specify=off  v_nominal_unit=V  v_nominal_value=1
  Phase Splitter : ee_lib/Connectors & References/Phase Splitter
      settings: SourceProductBaseCode=PS
  + : PMIOPort  Side=Left
  ~ : PMIOPort  Port=2  Side=Right
  - : PMIOPort  Port=3  Side=Left
  connections:
  Diode4/LConn1 -- Diode5/RConn1 -- Phase Splitter/RConn3
  -/RConn1 -- Diode3/LConn1 -- Diode5/LConn1 -- Diode1/LConn1
  Diode6/LConn1 -- Phase Splitter/RConn1 -- Diode1/RConn1
  Diode2/LConn1 -- Diode3/RConn1 -- Phase Splitter/RConn2
  ~/RConn1 -- Phase Splitter/LConn1
  Diode2/RConn1 -- Diode4/RConn1 -- +/RConn1 -- Diode6/RConn1

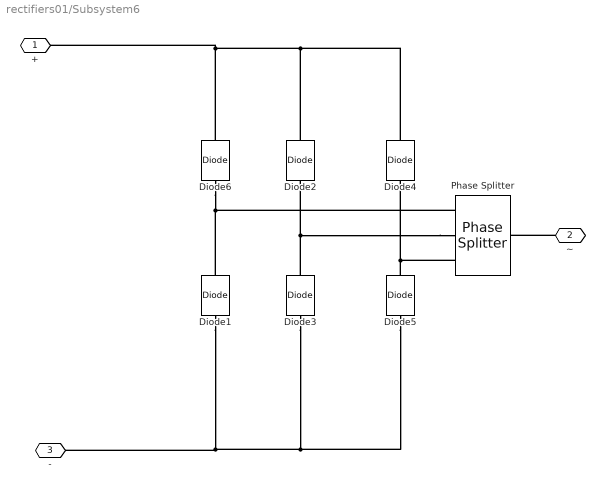
== system rectifiers01/Subsystem6 ==
  Diode{1..6} (6 alike) : fl_lib/Electrical/Electrical Elements/Diode  Vf=0.6 V  Ron=1e-5 Ohm  Goff=1e-8 1/Ohm  i_specify=off  i_priority=None  i=0 A  i_nominal_specify=off  i_nominal_unit=A  i_nominal_value=1  v_specify=off  v_priority=None  v=0 V  v_nominal_specify=off  v_nominal_unit=V  v_nominal_value=1
  Phase Splitter : ee_lib/Connectors & References/Phase Splitter
      settings: SourceProductBaseCode=PS
  + : PMIOPort  Side=Left
  ~ : PMIOPort  Port=2  Side=Right
  - : PMIOPort  Port=3  Side=Left
  connections:
  Diode6/RConn1 -- +/RConn1 -- Diode4/RConn1 -- Diode2/RConn1
  ~/RConn1 -- Phase Splitter/LConn1
  Phase Splitter/RConn2 -- Diode3/RConn1 -- Diode2/LConn1
  Diode1/RConn1 -- Phase Splitter/RConn1 -- Diode6/LConn1
  Diode1/LConn1 -- Diode5/LConn1 -- Diode3/LConn1 -- -/RConn1
  Phase Splitter/RConn3 -- Diode5/RConn1 -- Diode4/LConn1

== system rectifiers01/load ==
  Current Sensor : fl_lib/Electrical/Electrical Sensors/Current Sensor
  PS-Simulink Converter2 : nesl_utility/PS-Simulink Converter  PhysicalDomain=network_engine_domain  SubClassName=ps_output  LeftPortType=input  RightPortType=output  PseudoPeriodic=off  Frequencies=[]  Unit=inherit  AffineConversion=off
  PS-Simulink Converter3 : nesl_utility/PS-Simulink Converter  PhysicalDomain=network_engine_domain  SubClassName=ps_output  LeftPortType=input  RightPortType=output  PseudoPeriodic=off  Frequencies=[]  Unit=inherit  AffineConversion=off
  Resistor : fl_lib/Electrical/Electrical Elements/Resistor  R=R Ohm  i_specify=off  i_priority=None  i=0 A  i_nominal_specify=off  i_nominal_unit=A  i_nominal_value=1  v_specify=off  v_priority=None  v=0 V  v_nominal_specify=off  v_nominal_unit=V  v_nominal_value=1
  Terminator2 : Terminator
  Terminator3 : Terminator
  Voltage Sensor : fl_lib/Electrical/Electrical Sensors/Voltage Sensor
  + : PMIOPort  Side=Left
  - : PMIOPort  Port=2  Side=Right
  wires:
  PS-Simulink Converter3/1 -> Terminator3/1  "Idc1"
  PS-Simulink Converter2/1 -> Terminator2/1  "Vdc1"
  connections:
  +/RConn1 -- Current Sensor/LConn1
  Current Sensor/RConn2 -- Resistor/LConn1 -- Voltage Sensor/LConn1
  Voltage Sensor/RConn1 -- PS-Simulink Converter2/LConn1
  PS-Simulink Converter3/LConn1 -- Current Sensor/RConn1
  Voltage Sensor/RConn2 -- Resistor/RConn1 -- -/RConn1

== system rectifiers01/load  ==
  Current Sensor2 : fl_lib/Electrical/Electrical Sensors/Current Sensor
  PS-Simulink Converter10 : nesl_utility/PS-Simulink Converter  PhysicalDomain=network_engine_domain  SubClassName=ps_output  LeftPortType=input  RightPortType=output  PseudoPeriodic=off  Frequencies=[]  Unit=inherit  AffineConversion=off
  PS-Simulink Converter11 : nesl_utility/PS-Simulink Converter  PhysicalDomain=network_engine_domain  SubClassName=ps_output  LeftPortType=input  RightPortType=output  PseudoPeriodic=off  Frequencies=[]  Unit=inherit  AffineConversion=off
  Resistor : fl_lib/Electrical/Electrical Elements/Resistor  R=R Ohm  i_specify=off  i_priority=None  i=0 A  i_nominal_specify=off  i_nominal_unit=A  i_nominal_value=1  v_specify=off  v_priority=None  v=0 V  v_nominal_specify=off  v_nominal_unit=V  v_nominal_value=1
  Terminator10 : Terminator
  Terminator11 : Terminator
  Voltage Sensor2 : fl_lib/Electrical/Electrical Sensors/Voltage Sensor
  + : PMIOPort  Side=Left
  - : PMIOPort  Port=2  Side=Right
  wires:
  PS-Simulink Converter10/1 -> Terminator10/1  "Vdc3"
  PS-Simulink Converter11/1 -> Terminator11/1  "Idc3"
  connections:
  Current Sensor2/RConn2 -- Resistor/LConn1 -- Voltage Sensor2/LConn1
  PS-Simulink Converter11/LConn1 -- Current Sensor2/RConn1
  Voltage Sensor2/RConn1 -- PS-Simulink Converter10/LConn1
  Voltage Sensor2/RConn2 -- Resistor/RConn1 -- -/RConn1
  +/RConn1 -- Current Sensor2/LConn1

== system rectifiers01/load   ==
  Current Sensor1 : fl_lib/Electrical/Electrical Sensors/Current Sensor
  PS-Simulink Converter6 : nesl_utility/PS-Simulink Converter  PhysicalDomain=network_engine_domain  SubClassName=ps_output  LeftPortType=input  RightPortType=output  PseudoPeriodic=off  Frequencies=[]  Unit=inherit  AffineConversion=off
  PS-Simulink Converter7 : nesl_utility/PS-Simulink Converter  PhysicalDomain=network_engine_domain  SubClassName=ps_output  LeftPortType=input  RightPortType=output  PseudoPeriodic=off  Frequencies=[]  Unit=inherit  AffineConversion=off
  Resistor : fl_lib/Electrical/Electrical Elements/Resistor  R=R Ohm  i_specify=off  i_priority=None  i=0 A  i_nominal_specify=off  i_nominal_unit=A  i_nominal_value=1  v_specify=off  v_priority=None  v=0 V  v_nominal_specify=off  v_nominal_unit=V  v_nominal_value=1
  Terminator6 : Terminator
  Terminator7 : Terminator
  Voltage Sensor1 : fl_lib/Electrical/Electrical Sensors/Voltage Sensor
  + : PMIOPort  Side=Left
  - : PMIOPort  Port=2  Side=Right
  wires:
  PS-Simulink Converter6/1 -> Terminator6/1  "Vdc2"
  PS-Simulink Converter7/1 -> Terminator7/1  "Idc2"
  connections:
  Current Sensor1/RConn2 -- Resistor/LConn1 -- Voltage Sensor1/LConn1
  PS-Simulink Converter7/LConn1 -- Current Sensor1/RConn1
  Voltage Sensor1/RConn1 -- PS-Simulink Converter6/LConn1
  Voltage Sensor1/RConn2 -- Resistor/RConn1 -- -/RConn1
  +/RConn1 -- Current Sensor1/LConn1

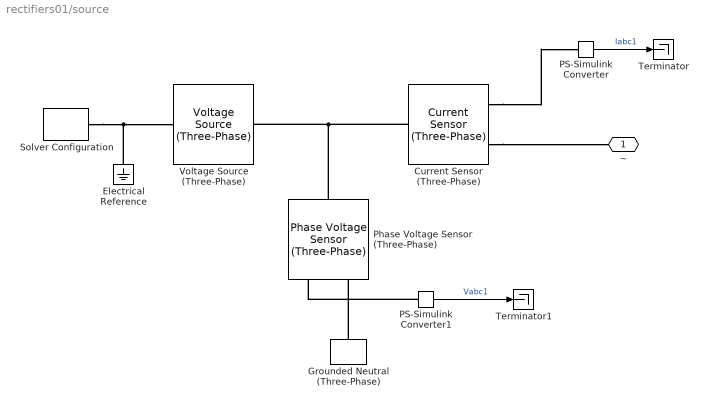
== system rectifiers01/source ==
  Current Sensor (Three-Phase) : ee_lib/Sensors & Transducers/Current Sensor (Three-Phase)
  Electrical Reference : fl_lib/Electrical/Electrical Elements/Electrical Reference
  Grounded Neutral (Three-Phase) : ee_lib/Connectors & References/Grounded Neutral (Three-Phase)
      settings: SourceProductBaseCode=PS
  PS-Simulink Converter : nesl_utility/PS-Simulink Converter  PhysicalDomain=network_engine_domain  SubClassName=ps_output  LeftPortType=input  RightPortType=output  PseudoPeriodic=off  Frequencies=[]  Unit=inherit  AffineConversion=off
  PS-Simulink Converter1 : nesl_utility/PS-Simulink Converter  PhysicalDomain=network_engine_domain  SubClassName=ps_output  LeftPortType=input  RightPortType=output  PseudoPeriodic=off  Frequencies=[]  Unit=inherit  AffineConversion=off
  Phase Voltage Sensor (Three-Phase) : ee_lib/Sensors & Transducers/Phase Voltage Sensor (Three-Phase)
      settings: SourceProductBaseCode=PS
  Solver Configuration : nesl_utility/Solver Configuration  PhysicalDomain=network_engine_domain  SubClassName=solver  LeftPortType=input  RightPortType=generic  Tones=[]  Harmonics=[]  SimulateNoise=off  Profile=off  UseLocalSampling=off  EnableSwitchedLinearOptims=on  FrequencyDomain=off  UseCCode=off  RelTol=0.001  AbsTol=1e-06  MinStep=1e-09  ToWorkspace=off  RevertToSquareIcSolve=off  NumHomotopyIterations=100  PhasorMode=off  PhasorModeNumHarmonics=1  DoDC=off  ResidualTolerance=1e-09  UseLocalSolver=on  LocalSolverChoice=NE_BACKWARD_EULER_ADVANCER  LocalSolverSampleTime=50e-6  DoFixedCost=on  MaxNonlinIter=3  MaxModeIter=2  ComputeImpulses=off  ImpulseIterations=2  LinearAlgebra=auto  EquationFormulation=NE_TIME_EF  DelaysMemoryBudget=1024  AutomaticFiltering=on  FilteringTimeConstant=0.001  PartitionStorageMethod=AS_NEEDED  PartitionMemoryBudget=1024  PartitionMethod=ROBUST
  Terminator : Terminator
  Terminator1 : Terminator
  Voltage Source (Three-Phase) : ee_lib/Sources/Voltage Source (Three-Phase)  vline_rms=sqrt(3) * 100 / sqrt(2) V  shift=0 deg  freq=60 Hz  impedance_option=0  SShortCircuit=1e6 V*A  XR=15  R=0.01 Ohm  L=3.97e-4 H  G_parasitic=0 1/Ohm  harmonic_option=0  harmonic_orders=[5, 7, 11, 13]  harmonic_ratios=[.1, .1, .1, .1]  I_specify=off  I_priority=None  I=[ 0 0 0 ] A  I_nominal_specify=off  I_nominal_unit=A  I_nominal_value=1
      settings: SourceProductBaseCode=PS
  ~ : PMIOPort  Side=Right
  wires:
  PS-Simulink Converter/1 -> Terminator/1  "Iabc1"
  PS-Simulink Converter1/1 -> Terminator1/1  "Vabc1"
  connections:
  PS-Simulink Converter1/LConn1 -- Phase Voltage Sensor (Three-Phase)/RConn1
  Grounded Neutral (Three-Phase)/LConn1 -- Phase Voltage Sensor (Three-Phase)/RConn2
  Current Sensor (Three-Phase)/RConn1 -- PS-Simulink Converter/LConn1
  Current Sensor (Three-Phase)/RConn2 -- ~/RConn1
  Electrical Reference/LConn1 -- Voltage Source (Three-Phase)/LConn1 -- Solver Configuration/RConn1
  Current Sensor (Three-Phase)/LConn1 -- Phase Voltage Sensor (Three-Phase)/LConn1 -- Voltage Source (Three-Phase)/RConn1

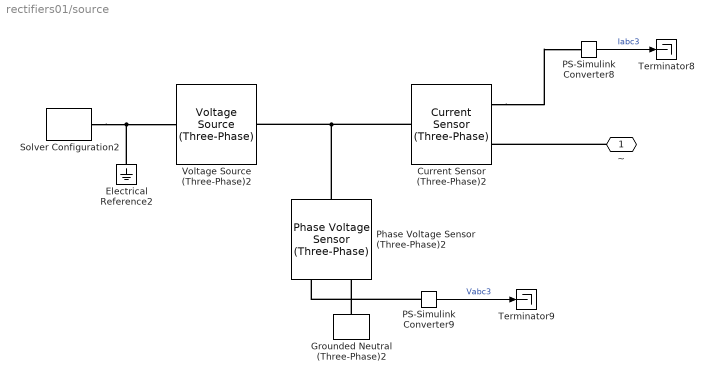
== system rectifiers01/source  ==
  Current Sensor (Three-Phase)2 : ee_lib/Sensors & Transducers/Current Sensor (Three-Phase)
  Electrical Reference2 : fl_lib/Electrical/Electrical Elements/Electrical Reference
  Grounded Neutral (Three-Phase)2 : ee_lib/Connectors & References/Grounded Neutral (Three-Phase)
      settings: SourceProductBaseCode=PS
  PS-Simulink Converter8 : nesl_utility/PS-Simulink Converter  PhysicalDomain=network_engine_domain  SubClassName=ps_output  LeftPortType=input  RightPortType=output  PseudoPeriodic=off  Frequencies=[]  Unit=inherit  AffineConversion=off
  PS-Simulink Converter9 : nesl_utility/PS-Simulink Converter  PhysicalDomain=network_engine_domain  SubClassName=ps_output  LeftPortType=input  RightPortType=output  PseudoPeriodic=off  Frequencies=[]  Unit=inherit  AffineConversion=off
  Phase Voltage Sensor (Three-Phase)2 : ee_lib/Sensors & Transducers/Phase Voltage Sensor (Three-Phase)
      settings: SourceProductBaseCode=PS
  Solver Configuration2 : nesl_utility/Solver Configuration  PhysicalDomain=network_engine_domain  SubClassName=solver  LeftPortType=input  RightPortType=generic  Tones=[]  Harmonics=[]  SimulateNoise=off  Profile=off  UseLocalSampling=off  EnableSwitchedLinearOptims=on  FrequencyDomain=off  UseCCode=off  RelTol=0.001  AbsTol=1e-06  MinStep=1e-09  ToWorkspace=off  RevertToSquareIcSolve=off  NumHomotopyIterations=100  PhasorMode=off  PhasorModeNumHarmonics=1  DoDC=off  ResidualTolerance=1e-09  UseLocalSolver=on  LocalSolverChoice=NE_BACKWARD_EULER_ADVANCER  LocalSolverSampleTime=50e-6  DoFixedCost=on  MaxNonlinIter=3  MaxModeIter=2  ComputeImpulses=off  ImpulseIterations=2  LinearAlgebra=auto  EquationFormulation=NE_TIME_EF  DelaysMemoryBudget=1024  AutomaticFiltering=on  FilteringTimeConstant=0.001  PartitionStorageMethod=AS_NEEDED  PartitionMemoryBudget=1024  PartitionMethod=ROBUST
  Terminator8 : Terminator
  Terminator9 : Terminator
  Voltage Source (Three-Phase)2 : ee_lib/Sources/Voltage Source (Three-Phase)  vline_rms=sqrt(3) * 100 / sqrt(2) V  shift=0 deg  freq=60 Hz  impedance_option=0  SShortCircuit=1e6 V*A  XR=15  R=0.01 Ohm  L=3.97e-4 H  G_parasitic=0 1/Ohm  harmonic_option=0  harmonic_orders=[5, 7, 11, 13]  harmonic_ratios=[.1, .1, .1, .1]  I_specify=off  I_priority=None  I=[ 0 0 0 ] A  I_nominal_specify=off  I_nominal_unit=A  I_nominal_value=1
      settings: SourceProductBaseCode=PS
  ~ : PMIOPort  Side=Right
  wires:
  PS-Simulink Converter8/1 -> Terminator8/1  "Iabc3"
  PS-Simulink Converter9/1 -> Terminator9/1  "Vabc3"
  connections:
  Current Sensor (Three-Phase)2/RConn1 -- PS-Simulink Converter8/LConn1
  Electrical Reference2/LConn1 -- Voltage Source (Three-Phase)2/LConn1 -- Solver Configuration2/RConn1
  Current Sensor (Three-Phase)2/LConn1 -- Phase Voltage Sensor (Three-Phase)2/LConn1 -- Voltage Source (Three-Phase)2/RConn1
  PS-Simulink Converter9/LConn1 -- Phase Voltage Sensor (Three-Phase)2/RConn1
  ~/RConn1 -- Current Sensor (Three-Phase)2/RConn2
  Grounded Neutral (Three-Phase)2/LConn1 -- Phase Voltage Sensor (Three-Phase)2/RConn2

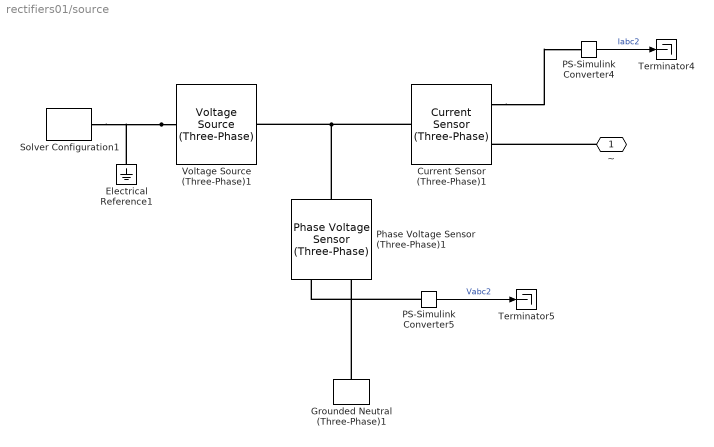
== system rectifiers01/source   ==
  Current Sensor (Three-Phase)1 : ee_lib/Sensors & Transducers/Current Sensor (Three-Phase)
  Electrical Reference1 : fl_lib/Electrical/Electrical Elements/Electrical Reference
  Grounded Neutral (Three-Phase)1 : ee_lib/Connectors & References/Grounded Neutral (Three-Phase)
      settings: SourceProductBaseCode=PS
  PS-Simulink Converter4 : nesl_utility/PS-Simulink Converter  PhysicalDomain=network_engine_domain  SubClassName=ps_output  LeftPortType=input  RightPortType=output  PseudoPeriodic=off  Frequencies=[]  Unit=inherit  AffineConversion=off
  PS-Simulink Converter5 : nesl_utility/PS-Simulink Converter  PhysicalDomain=network_engine_domain  SubClassName=ps_output  LeftPortType=input  RightPortType=output  PseudoPeriodic=off  Frequencies=[]  Unit=inherit  AffineConversion=off
  Phase Voltage Sensor (Three-Phase)1 : ee_lib/Sensors & Transducers/Phase Voltage Sensor (Three-Phase)
      settings: SourceProductBaseCode=PS
  Solver Configuration1 : nesl_utility/Solver Configuration  PhysicalDomain=network_engine_domain  SubClassName=solver  LeftPortType=input  RightPortType=generic  Tones=[]  Harmonics=[]  SimulateNoise=off  Profile=off  UseLocalSampling=off  EnableSwitchedLinearOptims=on  FrequencyDomain=off  UseCCode=off  RelTol=0.001  AbsTol=1e-06  MinStep=1e-09  ToWorkspace=off  RevertToSquareIcSolve=off  NumHomotopyIterations=100  PhasorMode=off  PhasorModeNumHarmonics=1  DoDC=off  ResidualTolerance=1e-09  UseLocalSolver=on  LocalSolverChoice=NE_BACKWARD_EULER_ADVANCER  LocalSolverSampleTime=50e-6  DoFixedCost=on  MaxNonlinIter=3  MaxModeIter=2  ComputeImpulses=off  ImpulseIterations=2  LinearAlgebra=auto  EquationFormulation=NE_TIME_EF  DelaysMemoryBudget=1024  AutomaticFiltering=on  FilteringTimeConstant=0.001  PartitionStorageMethod=AS_NEEDED  PartitionMemoryBudget=1024  PartitionMethod=ROBUST
  Terminator4 : Terminator
  Terminator5 : Terminator
  Voltage Source (Three-Phase)1 : ee_lib/Sources/Voltage Source (Three-Phase)  vline_rms=sqrt(3) * 100 / sqrt(2) V  shift=0 deg  freq=60 Hz  impedance_option=0  SShortCircuit=1e6 V*A  XR=15  R=0.01 Ohm  L=3.97e-4 H  G_parasitic=0 1/Ohm  harmonic_option=0  harmonic_orders=[5, 7, 11, 13]  harmonic_ratios=[.1, .1, .1, .1]  I_specify=off  I_priority=None  I=[ 0 0 0 ] A  I_nominal_specify=off  I_nominal_unit=A  I_nominal_value=1
      settings: SourceProductBaseCode=PS
  ~ : PMIOPort  Side=Right
  wires:
  PS-Simulink Converter4/1 -> Terminator4/1  "Iabc2"
  PS-Simulink Converter5/1 -> Terminator5/1  "Vabc2"
  connections:
  ~/RConn1 -- Current Sensor (Three-Phase)1/RConn2
  PS-Simulink Converter5/LConn1 -- Phase Voltage Sensor (Three-Phase)1/RConn1
  Phase Voltage Sensor (Three-Phase)1/LConn1 -- Current Sensor (Three-Phase)1/LConn1 -- Voltage Source (Three-Phase)1/RConn1
  Voltage Source (Three-Phase)1/LConn1 -- Electrical Reference1/LConn1 -- Solver Configuration1/RConn1
  Current Sensor (Three-Phase)1/RConn1 -- PS-Simulink Converter4/LConn1
  Grounded Neutral (Three-Phase)1/LConn1 -- Phase Voltage Sensor (Three-Phase)1/RConn2
